simulink model "xactive_rectifier_modified_CSVPWM_22march2025"  (R2024b)
settings: Solver=ode4  StartTime=0.0  StopTime=0.5  FixedStep=1e-6  RelTol=1e-3
values from neighbouring files (symbols this model uses):
  Cdc = 300e-6    (= 0.0003)    [ravi_active_rectifier.m]
  L = 2*Vm/(10000*pi*Ilrms)    (= 0.00173267748608)    [ravi_active_rectifier.m]
  MI = 2*sqrt(2)*Vnphrms/Vdc    [ravi_active_rectifier.m]
  MIL = 2*sqrt(2)*Vm/Vdc    [ravi_active_rectifier.m]
  R = Xl/10    (= 0.0544336686132)    [ravi_active_rectifier.m]
  Vdc = 700    [ravi_active_rectifier.m]
  Vm = 230    [ravi_active_rectifier.m]
libraries: spsIGBTDiodeLib x24, spsThreePhaseVIMeasurementLib x10, spsCurrentMeasurementLib x6, spsVoltageMeasurementLib x6, spsGroundLib x4, spsMeanLib x4, spsPower3phInstantaneousLib x4, simulink x4, spsThreePhaseSeriesRLCBranchLib x3, spsThreePhaseSourceLib x3, spsDCVoltageSourceLib x2, spsSeriesRLCBranchLib x2
settings Model: Creator=Atif iitb  LastModifiedBy=adity
settings DataIOCC: InspectSignalLogs=on  LoggingToFile=on

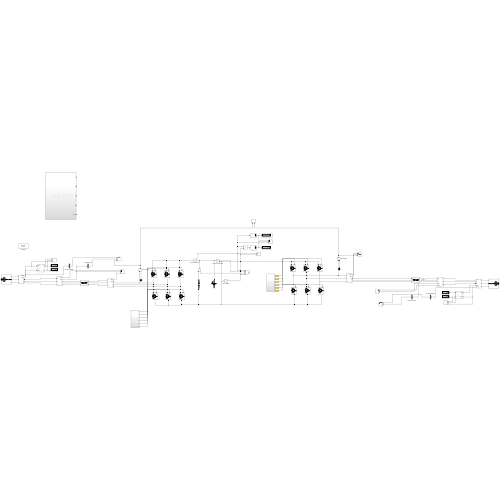
[thumbnail: Simulink's stored preview of the top-level diagram]
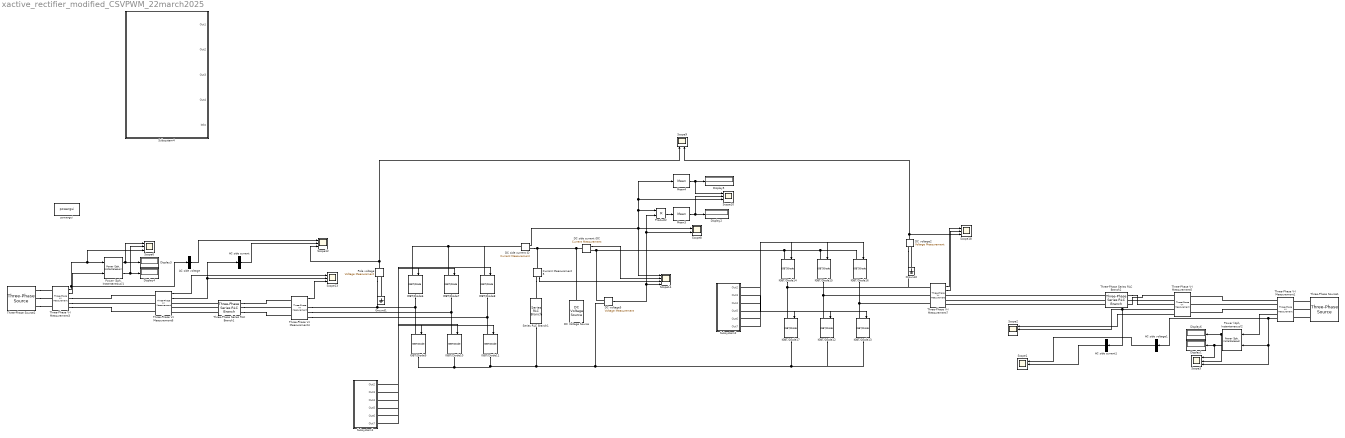
== system xactive_rectifier_modified_CSVPWM_22march2025 ==
  AC side current : Demux  Outputs=3
  AC side current1 : Demux  Outputs=3
  AC side voltage : Demux  Outputs=3
  AC side voltage1 : Demux  Outputs=3
  Current Measurement5 : spsCurrentMeasurementLib/Current Measurement  PhasorSimulation=off  OutputType=Complex  PSBequivalent=0
  DC Voltage Source : spsDCVoltageSourceLib/DC Voltage Source  Amplitude=Vdc  Measurements=None
  DC side current iD : spsCurrentMeasurementLib/Current Measurement  PhasorSimulation=off  OutputType=Complex  PSBequivalent=0
  DC side current iDC : spsCurrentMeasurementLib/Current Measurement  PhasorSimulation=off  OutputType=Complex  PSBequivalent=0
  DC voltage2 : spsVoltageMeasurementLib/Voltage Measurement  PhasorSimulation=off  OutputType=Complex  PSBequivalent=0
  DC voltage5 : spsVoltageMeasurementLib/Voltage Measurement  PhasorSimulation=off  OutputType=Complex  PSBequivalent=0
  Display{1..6} (6 alike) : Display
  Ground1 : spsGroundLib/Ground  LConnTagsString=a
  Ground2 : spsGroundLib/Ground  LConnTagsString=a
  IGBT/Diode{6..17} (12 alike) : spsIGBTDiodeLib/IGBT//Diode  Ron=1e-3  Rs=1e5  Cs=inf  Measurements=off
  Mean3 : spsMeanLib/Mean  Freq=50  Vinit=0  Ts=0
  Mean4 : spsMeanLib/Mean  Freq=50  Vinit=0  Ts=0
  Pole voltage : spsVoltageMeasurementLib/Voltage Measurement  PhasorSimulation=off  OutputType=Complex  PSBequivalent=0
  "Power (3ph, Instantaneous)1" : spsPower3phInstantaneousLib/Power (3ph, Instantaneous)
  "Power (3ph, Instantaneous)2" : spsPower3phInstantaneousLib/Power (3ph, Instantaneous)
  Product2 : Product
  Scope{1..3,6,10,12..13,18} (8 alike) : Scope  NumInputPorts=3
  Scope14 : Scope  NumInputPorts=4
  Scope8 : Scope  NumInputPorts=2
  Scope9 : Scope  NumInputPorts=2
  Series RLC Branch1 : spsSeriesRLCBranchLib/Series RLC Branch  LConnTagsString=__new0  RConnTagsString=__new0  BranchType=C  Resistance=1  Inductance=1e-3  SetiL0=off  InitialCurrent=0  Capacitance=Cdc  Setx0=off  InitialVoltage=0  Measurements=None
  Subsystem1 : Subsystem
  Subsystem2 : Subsystem
  Subsystem4 : Subsystem
  Three-Phase Series RLC Branch1 : spsThreePhaseSeriesRLCBranchLib/Three-Phase Series RLC Branch  LConnTagsString=A|B|C  RConnTagsString=A|B|C  BranchType=RL  Resistance=R  Inductance=L  Capacitance=1e-6  Measurements=None
  Three-Phase Series RLC Branch2 : spsThreePhaseSeriesRLCBranchLib/Three-Phase Series RLC Branch  LConnTagsString=A|B|C  RConnTagsString=A|B|C  BranchType=RL  Resistance=R  Inductance=L  Capacitance=1e-6  Measurements=None
  Three-Phase V-I Measurement1 : spsThreePhaseVIMeasurementLib/Three-Phase V-I Measurement  VoltageMeasurement=phase-to-ground  SetLabelV=off  LabelV=Vabc  Vpu=off  VpuLL=off  CurrentMeasurement=yes  SetLabelI=off  LabelI=Iabc  Ipu=off  Pbase=100e6  Vbase=500e3  OutputType=Complex  PhasorSimulation=off  PSBequivalent=0
  Three-Phase V-I Measurement3 : spsThreePhaseVIMeasurementLib/Three-Phase V-I Measurement  VoltageMeasurement=phase-to-ground  SetLabelV=off  LabelV=Vabc  Vpu=off  VpuLL=off  CurrentMeasurement=yes  SetLabelI=off  LabelI=Iabc  Ipu=off  Pbase=100e6  Vbase=500e3  OutputType=Complex  PhasorSimulation=off  PSBequivalent=0
  Three-Phase V-I Measurement4 : spsThreePhaseVIMeasurementLib/Three-Phase V-I Measurement  VoltageMeasurement=phase-to-phase  SetLabelV=off  LabelV=Vabc  Vpu=off  VpuLL=off  CurrentMeasurement=yes  SetLabelI=off  LabelI=Iabc  Ipu=off  Pbase=100e6  Vbase=500e3  OutputType=Complex  PhasorSimulation=off  PSBequivalent=0
  Three-Phase V-I Measurement5 : spsThreePhaseVIMeasurementLib/Three-Phase V-I Measurement  VoltageMeasurement=phase-to-phase  SetLabelV=off  LabelV=Vabc  Vpu=off  VpuLL=off  CurrentMeasurement=yes  SetLabelI=off  LabelI=Iabc  Ipu=off  Pbase=100e6  Vbase=500e3  OutputType=Complex  PhasorSimulation=off  PSBequivalent=0
  Three-Phase V-I Measurement6 : spsThreePhaseVIMeasurementLib/Three-Phase V-I Measurement  VoltageMeasurement=phase-to-phase  SetLabelV=off  LabelV=Vabc  Vpu=off  VpuLL=off  CurrentMeasurement=yes  SetLabelI=off  LabelI=Iabc  Ipu=off  Pbase=100e6  Vbase=500e3  OutputType=Complex  PhasorSimulation=off  PSBequivalent=0
  Three-Phase V-I Measurement7 : spsThreePhaseVIMeasurementLib/Three-Phase V-I Measurement  VoltageMeasurement=phase-to-ground  SetLabelV=off  LabelV=Vabc  Vpu=off  VpuLL=off  CurrentMeasurement=yes  SetLabelI=off  LabelI=Iabc  Ipu=off  Pbase=100e6  Vbase=500e3  OutputType=Complex  PhasorSimulation=off  PSBequivalent=0
  Three-Phase Source1 : spsThreePhaseSourceLib/Three-Phase Source  InternalConnection=Yg  VoltagePhases=off  Voltage=2.335782132615092e+02*sqrt(3)  PhaseAngle=0.890192885516744  Voltage_phases=[25e3 25e3 25e3]/sqrt(3)  PhaseAngles_phases=[0 -120 +120]  Frequency=50  NonIdealSource=off  SpecifyImpedance=off  Resistance=0.8929  Inductance=16.58e-3  ShortCircuitLevel=100e6  BaseVoltage=25e3  XRratio=7  BusType=swing  Pref=10e3  Qref=0  Prefabc=[10e3, 10e3, 10e3]  Qrefabc=[0, 0, 0]  Qmin=-inf  Qmax=inf
  Three-Phase Source2 : spsThreePhaseSourceLib/Three-Phase Source  InternalConnection=Yg  VoltagePhases=off  Voltage=Vm*sqrt(3)  PhaseAngle=Delta  Voltage_phases=[25e3 25e3 25e3]/sqrt(3)  PhaseAngles_phases=[0 -120 +120]  Frequency=50  NonIdealSource=off  SpecifyImpedance=off  Resistance=0.8929  Inductance=16.58e-3  ShortCircuitLevel=100e6  BaseVoltage=25e3  XRratio=7  BusType=swing  Pref=10e3  Qref=0  Prefabc=[10e3, 10e3, 10e3]  Qrefabc=[0, 0, 0]  Qmin=-inf  Qmax=inf
  powergui : sps_lib/powergui  Priority=1  SimulationMode=Discrete  SampleTime=1e-6  frequency=60  Iterations=50  frequencyindice=0  Pbase=100e6  ErrMax=1e-4  UnitsV=kV  UnitsW=MW  buscounter=0  FunctionMessages=off  echomessages=off  EnableUseOfTLC=off  CurrentSourceSwitches=off  DisableSnubberDevices=off  DisableRonSwitches=off  DisableVfSwitches=off  DisplayEquations=off  AutomaticDiscreteSolvers=off  SolverType=Tustin/Backward Euler (TBE)  Interpol=off  ExternalGateDelay=off  methode=off  Ts=100  x0status=blocks  SPID=on  SwTol=0  HookPort=off  NonlinearTolerance=1e-4  nMaxIteration=100  ContinueOnMaxIteration=off  RestoreLinks=warning  ResistiveCurrentMeasurement=off  Frange=[0:2:500]  Ylog=off  Xlog=on  ShowGrid=off  save=off  variable=ZData  structure=0  ZoomFFT=off  StartTime=0.0  cycles=1  DisplayStyle=1  fundamental=60  FreqAxis=off  MaxFrequency=1000  frequencyindicesteady=1  RmsSteady=1  display=off
  wires:
  Subsystem1/2(Out3) -> IGBT/Diode9/1
  Subsystem1/6(Out7) -> IGBT/Diode11/1
  Mean4/1 -> Scope10/1, Display5/1
  Subsystem1/3(Out4) -> IGBT/Diode7/1
  DC side current iD/1 -> Scope14/1, Mean4/1, Scope10/3, Product2/1, Scope8/1
  Subsystem1/5(Out6) -> IGBT/Diode8/1
  AC side current/2 -> Scope12/2
  Mean3/1 -> Scope10/2, Display2/1
  Three-Phase V-I Measurement6/2 -> Scope13/2, AC side current/1
  Product2/1 -> Mean3/1
  Three-Phase V-I Measurement4/1 -> Scope13/3
  Subsystem1/1(Out2) -> IGBT/Diode6/1
  Pole voltage/1 -> Scope12/3, Scope9/1
  Three-Phase V-I Measurement6/1 -> Scope13/1
  Subsystem1/4(Out5) -> IGBT/Diode10/1
  Three-Phase V-I Measurement3/1 -> AC side voltage/1, Scope6/3, "Power (3ph, Instantaneous)1"/1
  Three-Phase V-I Measurement3/2 -> "Power (3ph, Instantaneous)1"/2
  "Power (3ph, Instantaneous)1"/1 -> Scope6/1, Display3/1
  "Power (3ph, Instantaneous)1"/2 -> Scope6/2, Display4/1
  AC side voltage/2 -> Scope12/1
  DC voltage5/1 -> Scope8/2, Product2/2, Scope14/4
  Current Measurement5/1 -> Scope14/3
  DC side current iDC/1 -> Scope14/2
  Subsystem2/1(Out2) -> IGBT/Diode14/1
  Subsystem2/2(Out3) -> IGBT/Diode17/1
  Subsystem2/3(Out4) -> IGBT/Diode15/1
  Subsystem2/4(Out5) -> IGBT/Diode12/1
  Subsystem2/5(Out6) -> IGBT/Diode16/1
  Subsystem2/6(Out7) -> IGBT/Diode13/1
  Three-Phase V-I Measurement7/2 -> Scope18/2
  Three-Phase V-I Measurement7/1 -> Scope18/1
  DC voltage2/1 -> Scope18/3, Scope9/2
  AC side voltage1/2 -> Scope1/1
  Three-Phase V-I Measurement1/1 -> Scope3/3, "Power (3ph, Instantaneous)2"/1, AC side voltage1/1
  "Power (3ph, Instantaneous)2"/2 -> Scope3/2, Display6/1
  Three-Phase V-I Measurement1/2 -> "Power (3ph, Instantaneous)2"/2
  AC side current1/2 -> Scope1/2
  Three-Phase V-I Measurement5/1 -> Scope2/1
  Three-Phase V-I Measurement5/2 -> Scope2/2, AC side current1/1
  "Power (3ph, Instantaneous)2"/1 -> Scope3/1, Display1/1
  connections:
  Pole voltage/LConn1 -- Three-Phase V-I Measurement4/RConn1 -- IGBT/Diode6/RConn1 -- IGBT/Diode9/LConn1
  IGBT/Diode6/LConn1 -- IGBT/Diode7/LConn1 -- IGBT/Diode8/LConn1 -- DC side current iD/LConn1
  Three-Phase V-I Measurement4/RConn2 -- IGBT/Diode7/RConn1 -- IGBT/Diode10/LConn1
  Three-Phase V-I Measurement4/RConn3 -- IGBT/Diode8/RConn1 -- IGBT/Diode11/LConn1
  Three-Phase Series RLC Branch1/RConn1 -- Three-Phase V-I Measurement4/LConn1
  Three-Phase Series RLC Branch1/LConn1 -- Three-Phase V-I Measurement6/RConn1
  Three-Phase Series RLC Branch1/RConn2 -- Three-Phase V-I Measurement4/LConn2
  Three-Phase Series RLC Branch1/RConn3 -- Three-Phase V-I Measurement4/LConn3
  Three-Phase Series RLC Branch1/LConn2 -- Three-Phase V-I Measurement6/RConn2
  Three-Phase Series RLC Branch1/LConn3 -- Three-Phase V-I Measurement6/RConn3
  Three-Phase Source2/RConn1 -- Three-Phase V-I Measurement3/LConn1
  Three-Phase Source2/RConn2 -- Three-Phase V-I Measurement3/LConn2
  Three-Phase Source2/RConn3 -- Three-Phase V-I Measurement3/LConn3
  Three-Phase V-I Measurement3/RConn1 -- Three-Phase V-I Measurement6/LConn1
  Three-Phase V-I Measurement3/RConn2 -- Three-Phase V-I Measurement6/LConn2
  Three-Phase V-I Measurement3/RConn3 -- Three-Phase V-I Measurement6/LConn3
  Current Measurement5/RConn1 -- Series RLC Branch1/LConn1
  DC side current iD/RConn1 -- Current Measurement5/LConn1 -- DC Voltage Source/RConn1 -- DC side current iDC/LConn1
  IGBT/Diode15/RConn1 -- Three-Phase V-I Measurement7/LConn2 -- IGBT/Diode12/LConn1
  IGBT/Diode14/RConn1 -- DC voltage2/LConn1 -- Three-Phase V-I Measurement7/LConn1 -- IGBT/Diode17/LConn1
  IGBT/Diode16/RConn1 -- Three-Phase V-I Measurement7/LConn3 -- IGBT/Diode13/LConn1
  DC side current iDC/RConn1 -- IGBT/Diode14/LConn1 -- IGBT/Diode15/LConn1 -- IGBT/Diode16/LConn1 -- DC voltage5/LConn1
  Ground1/LConn1 -- Pole voltage/LConn2
  Ground2/LConn1 -- DC voltage2/LConn2
  IGBT/Diode9/RConn1 -- Series RLC Branch1/RConn1 -- IGBT/Diode12/RConn1 -- IGBT/Diode13/RConn1 -- IGBT/Diode17/RConn1 -- DC voltage5/LConn2 -- IGBT/Diode11/RConn1 -- IGBT/Diode10/RConn1
  Three-Phase Series RLC Branch2/LConn2 -- Three-Phase V-I Measurement5/RConn2
  Three-Phase Source1/RConn3 -- Three-Phase V-I Measurement1/LConn3
  Three-Phase Source1/RConn1 -- Three-Phase V-I Measurement1/LConn1
  Three-Phase Source1/RConn2 -- Three-Phase V-I Measurement1/LConn2
  Three-Phase Series RLC Branch2/LConn1 -- Three-Phase V-I Measurement5/RConn1
  Three-Phase V-I Measurement1/RConn3 -- Three-Phase V-I Measurement5/LConn3
  Three-Phase V-I Measurement1/RConn1 -- Three-Phase V-I Measurement5/LConn1
  Three-Phase Series RLC Branch2/LConn3 -- Three-Phase V-I Measurement5/RConn3
  Three-Phase V-I Measurement1/RConn2 -- Three-Phase V-I Measurement5/LConn2
  Three-Phase Series RLC Branch2/RConn1 -- Three-Phase V-I Measurement7/RConn1
  Three-Phase Series RLC Branch2/RConn2 -- Three-Phase V-I Measurement7/RConn2
  Three-Phase Series RLC Branch2/RConn3 -- Three-Phase V-I Measurement7/RConn3

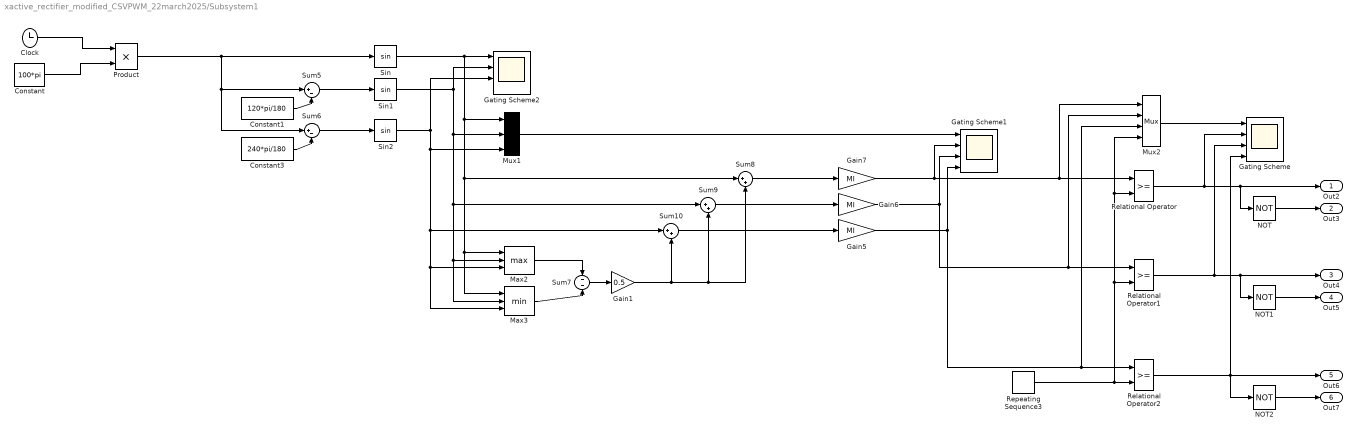
== system xactive_rectifier_modified_CSVPWM_22march2025/Subsystem1 ==
  Clock : Clock
  Constant : Constant  Value=100*pi
  Constant1 : Constant  Value=120*pi/180
  Constant3 : Constant  Value=240*pi/180
  Gain1 : Gain  Gain=0.5
  Gain5 : Gain  Gain=MI
  Gain6 : Gain  Gain=MI
  Gain7 : Gain  Gain=MI
  Gating Scheme : Scope  NumInputPorts=4
  Gating Scheme1 : Scope  NumInputPorts=4
  Gating Scheme2 : Scope  NumInputPorts=4
  Max2 : MinMax  Function=max  Inputs=3
  Max3 : MinMax  Inputs=3
  Mux1 : Mux  Inputs=3.
  Mux2 : Mux
  NOT : Logic  Operator=NOT  IconShape=distinctive  AllPortsSameDT=off  OutDataTypeStr=boolean
  NOT1 : Logic  Operator=NOT  IconShape=distinctive  AllPortsSameDT=off  OutDataTypeStr=boolean
  NOT2 : Logic  Operator=NOT  IconShape=distinctive  AllPortsSameDT=off  OutDataTypeStr=boolean
  Product : Product
  Relational Operator : RelationalOperator  OutDataTypeStr=boolean  RndMeth=Simplest  InputSameDT=off
  Relational Operator1 : RelationalOperator  OutDataTypeStr=boolean  RndMeth=Simplest  InputSameDT=off
  Relational Operator2 : RelationalOperator  OutDataTypeStr=boolean  RndMeth=Simplest  InputSameDT=off
  Repeating Sequence3 : simulink/Sources/Repeating Sequence  rep_seq_t=[0 1 2]*[1/40000]  rep_seq_y=[-1 1 -1]
  Sin : Trigonometry
  Sin1 : Trigonometry
  Sin2 : Trigonometry
  Sum10 : Sum  Inputs=|++
  Sum5 : Sum  Inputs=|+-
  Sum6 : Sum  Inputs=|+-
  Sum7 : Sum  Inputs=--
  Sum8 : Sum  Inputs=|++
  Sum9 : Sum  Inputs=|++
  Out2 : Outport
  Out3 : Outport  Port=2
  Out4 : Outport  Port=3
  Out5 : Outport  Port=4
  Out6 : Outport  Port=5
  Out7 : Outport  Port=6
  wires:
  NOT2/1 -> Out7/1
  Constant/1 -> Product/2
  Constant1/1 -> Sum5/2
  Sin/1 -> Gating Scheme2/1, Sum8/1, Max2/1, Max3/1, Mux1/1
  Relational Operator2/1 -> Out6/1, Gating Scheme/4, NOT2/1
  Sum10/1 -> Gain5/1
  NOT/1 -> Out3/1
  Relational Operator/1 -> Out2/1, NOT/1, Gating Scheme/2
  Sum9/1 -> Gain6/1
  Sum5/1 -> Sin1/1
  Product/1 -> Sin/1, Sum6/1, Sum5/1
  Mux2/1 -> Gating Scheme/1
  Sin2/1 -> Sum10/1, Max3/3, Max2/3, Mux1/3, Gating Scheme2/3
  Sin1/1 -> Max3/2, Max2/2, Sum9/1, Mux1/2, Gating Scheme2/2
  Clock/1 -> Product/1
  Repeating Sequence3/1 -> Relational Operator1/2, Mux2/4, Relational Operator/2, Relational Operator2/2
  Relational Operator1/1 -> Out4/1, NOT1/1, Gating Scheme/3
  Max2/1 -> Sum7/1
  Sum7/1 -> Gain1/1
  Max3/1 -> Sum7/2
  Constant3/1 -> Sum6/2
  Sum6/1 -> Sin2/1
  NOT1/1 -> Out5/1
  Mux1/1 -> Gating Scheme1/1
  Gain1/1 -> Sum10/2, Sum9/2, Sum8/2
  Sum8/1 -> Gain7/1
  Gain7/1 -> Gating Scheme1/2, Mux2/1, Relational Operator/1
  Gain6/1 -> Mux2/2, Relational Operator1/1, Gating Scheme1/3
  Gain5/1 -> Mux2/3, Relational Operator2/1, Gating Scheme1/4

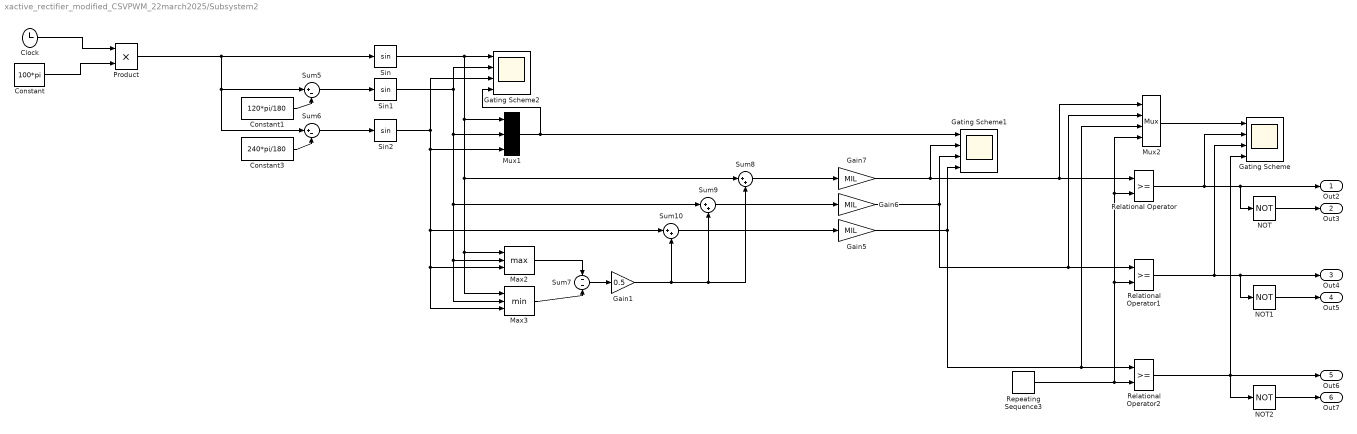
== system xactive_rectifier_modified_CSVPWM_22march2025/Subsystem2 ==
  Clock : Clock
  Constant : Constant  Value=100*pi
  Constant1 : Constant  Value=120*pi/180
  Constant3 : Constant  Value=240*pi/180
  Gain1 : Gain  Gain=0.5
  Gain5 : Gain  Gain=MIL
  Gain6 : Gain  Gain=MIL
  Gain7 : Gain  Gain=MIL
  Gating Scheme : Scope  NumInputPorts=4
  Gating Scheme1 : Scope  NumInputPorts=4
  Gating Scheme2 : Scope  NumInputPorts=4
  Max2 : MinMax  Function=max  Inputs=3
  Max3 : MinMax  Inputs=3
  Mux1 : Mux  Inputs=3.
  Mux2 : Mux
  NOT : Logic  Operator=NOT  IconShape=distinctive  AllPortsSameDT=off  OutDataTypeStr=boolean
  NOT1 : Logic  Operator=NOT  IconShape=distinctive  AllPortsSameDT=off  OutDataTypeStr=boolean
  NOT2 : Logic  Operator=NOT  IconShape=distinctive  AllPortsSameDT=off  OutDataTypeStr=boolean
  Product : Product
  Relational Operator : RelationalOperator  OutDataTypeStr=boolean  RndMeth=Simplest  InputSameDT=off
  Relational Operator1 : RelationalOperator  OutDataTypeStr=boolean  RndMeth=Simplest  InputSameDT=off
  Relational Operator2 : RelationalOperator  OutDataTypeStr=boolean  RndMeth=Simplest  InputSameDT=off
  Repeating Sequence3 : simulink/Sources/Repeating Sequence  rep_seq_t=[0 1 2]*[1/40000]  rep_seq_y=[-1 1 -1]
  Sin : Trigonometry
  Sin1 : Trigonometry
  Sin2 : Trigonometry
  Sum10 : Sum  Inputs=|++
  Sum5 : Sum  Inputs=|+-
  Sum6 : Sum  Inputs=|+-
  Sum7 : Sum  Inputs=--
  Sum8 : Sum  Inputs=|++
  Sum9 : Sum  Inputs=|++
  Out2 : Outport
  Out3 : Outport  Port=2
  Out4 : Outport  Port=3
  Out5 : Outport  Port=4
  Out6 : Outport  Port=5
  Out7 : Outport  Port=6
  wires:
  Gain5/1 -> Gating Scheme1/4, Relational Operator2/1, Mux2/3
  Gain6/1 -> Gating Scheme1/3, Relational Operator1/1, Mux2/2
  Gain7/1 -> Relational Operator/1, Mux2/1, Gating Scheme1/2
  Sum8/1 -> Gain7/1
  Gain1/1 -> Sum8/2, Sum9/2, Sum10/2
  Mux1/1 -> Gating Scheme2/4, Gating Scheme1/1
  NOT1/1 -> Out5/1
  Sum6/1 -> Sin2/1
  Constant3/1 -> Sum6/2
  Max3/1 -> Sum7/2
  Sum7/1 -> Gain1/1
  Max2/1 -> Sum7/1
  Relational Operator1/1 -> Gating Scheme/3, NOT1/1, Out4/1
  Repeating Sequence3/1 -> Relational Operator2/2, Relational Operator/2, Mux2/4, Relational Operator1/2
  Clock/1 -> Product/1
  Sin1/1 -> Gating Scheme2/2, Mux1/2, Sum9/1, Max2/2, Max3/2
  Sin2/1 -> Gating Scheme2/3, Mux1/3, Max2/3, Max3/3, Sum10/1
  Mux2/1 -> Gating Scheme/1
  Product/1 -> Sum5/1, Sum6/1, Sin/1
  Sum5/1 -> Sin1/1
  Sum9/1 -> Gain6/1
  Relational Operator/1 -> Gating Scheme/2, NOT/1, Out2/1
  NOT/1 -> Out3/1
  Sum10/1 -> Gain5/1
  Relational Operator2/1 -> NOT2/1, Gating Scheme/4, Out6/1
  Sin/1 -> Mux1/1, Max3/1, Max2/1, Sum8/1, Gating Scheme2/1
  Constant1/1 -> Sum5/2
  Constant/1 -> Product/2
  NOT2/1 -> Out7/1

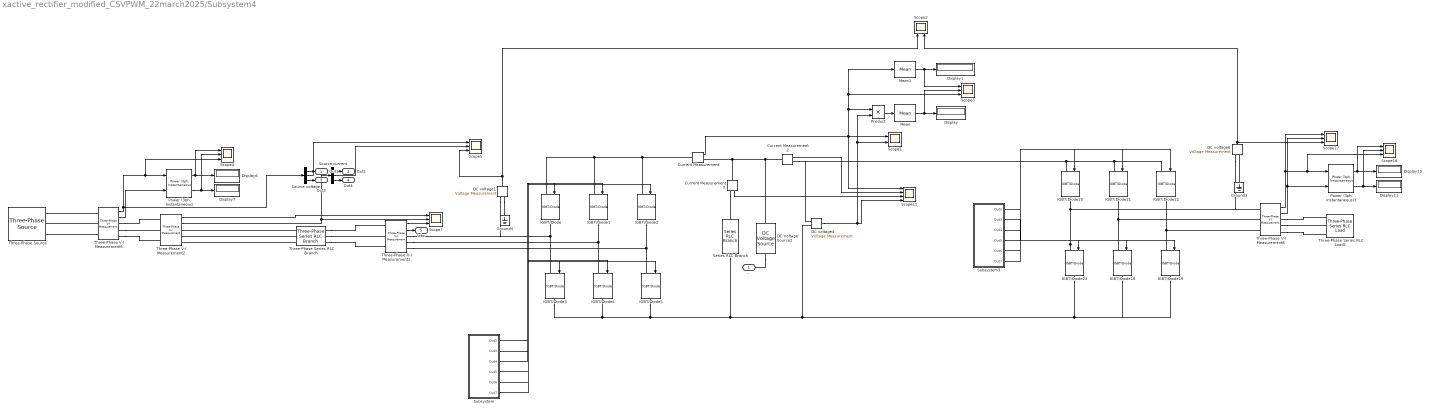
== system xactive_rectifier_modified_CSVPWM_22march2025/Subsystem4 ==
  Current Measurement : spsCurrentMeasurementLib/Current Measurement  PhasorSimulation=off  OutputType=Complex  PSBequivalent=0
  Current Measurement2 : spsCurrentMeasurementLib/Current Measurement  PhasorSimulation=off  OutputType=Complex  PSBequivalent=0
  Current Measurement3 : spsCurrentMeasurementLib/Current Measurement  PhasorSimulation=off  OutputType=Complex  PSBequivalent=0
  DC Voltage Source2 : spsDCVoltageSourceLib/DC Voltage Source  Amplitude=Vdc  Measurements=None
  DC voltage1 : spsVoltageMeasurementLib/Voltage Measurement  PhasorSimulation=off  OutputType=Complex  PSBequivalent=0
  DC voltage4 : spsVoltageMeasurementLib/Voltage Measurement  PhasorSimulation=off  OutputType=Complex  PSBequivalent=0
  DC voltage6 : spsVoltageMeasurementLib/Voltage Measurement  PhasorSimulation=off  OutputType=Complex  PSBequivalent=0
  Display{,1,6..7,10..11} (6 alike) : Display
  Ground3 : spsGroundLib/Ground  LConnTagsString=a
  Ground4 : spsGroundLib/Ground  LConnTagsString=a
  IGBT/Diode{,1..5,18..23} (12 alike) : spsIGBTDiodeLib/IGBT//Diode  Ron=1e-3  Rs=1e5  Cs=inf  Measurements=off
  Mean : spsMeanLib/Mean  Freq=50  Vinit=0  Ts=0
  Mean1 : spsMeanLib/Mean  Freq=50  Vinit=0  Ts=0
  "Power (3ph, Instantaneous)" : spsPower3phInstantaneousLib/Power (3ph, Instantaneous)
  "Power (3ph, Instantaneous)3" : spsPower3phInstantaneousLib/Power (3ph, Instantaneous)
  Product : Product
  Scope1 : Scope  NumInputPorts=2
  Scope11 : Scope  NumInputPorts=4
  Scope{3..5,7,16..17} (6 alike) : Scope  NumInputPorts=3
  Scope2 : Scope  NumInputPorts=2
  Series RLC Branch : spsSeriesRLCBranchLib/Series RLC Branch  LConnTagsString=__new0  RConnTagsString=__new0  BranchType=C  Resistance=1  Inductance=1e-3  SetiL0=off  InitialCurrent=0  Capacitance=Cdc  Setx0=off  InitialVoltage=0  Measurements=None
  Source current : Demux  Outputs=3
  Source voltage : Demux  Outputs=3
  Subsystem : Subsystem
  Subsystem3 : Subsystem
  Three-Phase Series RLC Branch : spsThreePhaseSeriesRLCBranchLib/Three-Phase Series RLC Branch  LConnTagsString=A|B|C  RConnTagsString=A|B|C  BranchType=RL  Resistance=R  Inductance=L  Capacitance=1e-6  Measurements=None
  Three-Phase Series RLC Load1 : spsThreePhaseSeriesRLCLoadLib/Three-Phase Series RLC Load  LConnTagsString=A|B|C  Configuration=Y (grounded)  NominalVoltage=230*sqrt(3)  Vabc=[1e3 1e3 1e3]  Vabcp=[1e3 1e3 1e3]  NominalFrequency=50  UnbalancedPower=off  ActivePower=0  InductivePower=QL  CapacitivePower=0  Pabc=[10e3 9e3 11e3]  QLabc=[100 90 110]  QCabc=[100 90 110]  Pabcp=[10e3 9e3 11e3]  QLabcp=[100 90 110]  QCabcp=[100 90 110]  Measurements=None  LoadType=constant Z
  Three-Phase V-I Measurement{1..2,5,8} (4 alike) : spsThreePhaseVIMeasurementLib/Three-Phase V-I Measurement  VoltageMeasurement=phase-to-ground  SetLabelV=off  LabelV=Vabc  Vpu=off  VpuLL=off  CurrentMeasurement=yes  SetLabelI=off  LabelI=Iabc  Ipu=off  Pbase=100e6  Vbase=500e3  OutputType=Complex  PhasorSimulation=off  PSBequivalent=0
  Three-Phase Source : spsThreePhaseSourceLib/Three-Phase Source  InternalConnection=Yg  VoltagePhases=off  Voltage=Vm*sqrt(3)  PhaseAngle=Delta  Voltage_phases=[25e3 25e3 25e3]/sqrt(3)  PhaseAngles_phases=[0 -120 +120]  Frequency=50  NonIdealSource=off  SpecifyImpedance=off  Resistance=0.8929  Inductance=16.58e-3  ShortCircuitLevel=100e6  BaseVoltage=25e3  XRratio=7  BusType=swing  Pref=10e3  Qref=0  Prefabc=[10e3, 10e3, 10e3]  Qrefabc=[0, 0, 0]  Qmin=-inf  Qmax=inf
  - : PMIOPort  Side=Left
  Out1 : Outport
  Out2 : Outport  Port=2
  Out3 : Outport  Port=3
  Out4 : Outport  Port=4
  Iabc : Outport  Port=5
  wires:
  Subsystem/4(Out5) -> IGBT/Diode4/1
  Subsystem/5(Out6) -> IGBT/Diode2/1
  Current Measurement/1 -> Scope11/1, Mean1/1, Scope3/3, Product/1, Scope1/1
  "Power (3ph, Instantaneous)3"/1 -> Display10/1, Scope16/1
  DC voltage6/1 -> Scope2/2, Scope17/3
  Three-Phase V-I Measurement2/1 -> Scope7/1
  Subsystem3/2(Out3) -> IGBT/Diode23/1
  Source voltage/2 -> Scope5/1
  Current Measurement2/1 -> Scope11/2
  Subsystem3/6(Out7) -> IGBT/Diode19/1
  Subsystem/3(Out4) -> IGBT/Diode1/1
  Three-Phase V-I Measurement5/1 -> Source voltage/1, Scope4/3, "Power (3ph, Instantaneous)"/1
  Subsystem/1(Out2) -> IGBT/Diode/1
  Three-Phase V-I Measurement8/1 -> Scope17/1, "Power (3ph, Instantaneous)3"/1, Scope16/3
  Three-Phase V-I Measurement2/2 -> Source current/1, Scope7/2
  Three-Phase V-I Measurement8/2 -> Scope17/2, "Power (3ph, Instantaneous)3"/2
  Subsystem3/4(Out5) -> IGBT/Diode18/1
  Mean1/1 -> Scope3/1, Display1/1
  Product/1 -> Mean/1
  "Power (3ph, Instantaneous)3"/2 -> Display11/1, Scope16/2
  Three-Phase V-I Measurement5/2 -> "Power (3ph, Instantaneous)"/2
  Three-Phase V-I Measurement1/2 -> Iabc/1
  Source current/2 -> Scope5/2
  Subsystem/6(Out7) -> IGBT/Diode5/1
  Subsystem3/5(Out6) -> IGBT/Diode22/1
  Source voltage/1 -> Out1/1
  DC voltage1/1 -> Scope5/3, Scope2/1
  Subsystem3/3(Out4) -> IGBT/Diode21/1
  "Power (3ph, Instantaneous)"/1 -> Scope4/1, Display6/1
  Subsystem/2(Out3) -> IGBT/Diode3/1
  Subsystem3/1(Out2) -> IGBT/Diode20/1
  Three-Phase V-I Measurement1/1 -> Scope7/3
  Current Measurement3/1 -> Scope11/3
  "Power (3ph, Instantaneous)"/2 -> Scope4/2, Display7/1
  DC voltage4/1 -> Product/2, Scope1/2, Scope11/4
  Mean/1 -> Scope3/2, Display/1
  Source current/1 -> Out2/1
  Source voltage/3 -> Out3/1
  Source current/3 -> Out4/1
  connections:
  Current Measurement3/LConn1 -- Current Measurement2/LConn1 -- DC Voltage Source2/RConn1 -- Current Measurement/RConn1
  IGBT/Diode22/RConn1 -- Three-Phase V-I Measurement8/LConn3 -- IGBT/Diode19/LConn1
  Three-Phase V-I Measurement5/RConn2 -- Three-Phase V-I Measurement2/LConn2
  Three-Phase V-I Measurement8/RConn2 -- Three-Phase Series RLC Load1/LConn2
  IGBT/Diode5/RConn1 -- Series RLC Branch/RConn1 -- IGBT/Diode23/RConn1 -- IGBT/Diode18/RConn1 -- IGBT/Diode19/RConn1 -- DC voltage4/LConn2 -- IGBT/Diode4/RConn1 -- IGBT/Diode3/RConn1
  Three-Phase V-I Measurement5/RConn3 -- Three-Phase V-I Measurement2/LConn3
  Three-Phase V-I Measurement5/LConn3 -- Three-Phase Source/RConn3
  Three-Phase Series RLC Branch/RConn2 -- Three-Phase V-I Measurement1/LConn2
  IGBT/Diode2/LConn1 -- IGBT/Diode/LConn1 -- IGBT/Diode1/LConn1 -- Current Measurement/LConn1
  IGBT/Diode20/LConn1 -- DC voltage4/LConn1 -- Current Measurement2/RConn1 -- IGBT/Diode21/LConn1 -- IGBT/Diode22/LConn1
  DC voltage1/LConn2 -- Ground4/LConn1
  DC Voltage Source2/LConn1 -- -/RConn1
  IGBT/Diode/RConn1 -- Three-Phase V-I Measurement1/RConn1 -- DC voltage1/LConn1 -- IGBT/Diode3/LConn1
  Three-Phase V-I Measurement8/RConn3 -- Three-Phase Series RLC Load1/LConn3
  Three-Phase V-I Measurement5/LConn2 -- Three-Phase Source/RConn2
  IGBT/Diode1/RConn1 -- Three-Phase V-I Measurement1/RConn2 -- IGBT/Diode4/LConn1
  Three-Phase Series RLC Branch/LConn3 -- Three-Phase V-I Measurement2/RConn3
  IGBT/Diode23/LConn1 -- DC voltage6/LConn1 -- Three-Phase V-I Measurement8/LConn1 -- IGBT/Diode20/RConn1
  Three-Phase V-I Measurement8/RConn1 -- Three-Phase Series RLC Load1/LConn1
  Three-Phase V-I Measurement5/LConn1 -- Three-Phase Source/RConn1
  Three-Phase Series RLC Branch/LConn2 -- Three-Phase V-I Measurement2/RConn2
  Three-Phase V-I Measurement5/RConn1 -- Three-Phase V-I Measurement2/LConn1
  Three-Phase Series RLC Branch/RConn1 -- Three-Phase V-I Measurement1/LConn1
  Current Measurement3/RConn1 -- Series RLC Branch/LConn1
  Three-Phase Series RLC Branch/RConn3 -- Three-Phase V-I Measurement1/LConn3
  IGBT/Diode21/RConn1 -- Three-Phase V-I Measurement8/LConn2 -- IGBT/Diode18/LConn1
  Ground3/LConn1 -- DC voltage6/LConn2
  IGBT/Diode2/RConn1 -- Three-Phase V-I Measurement1/RConn3 -- IGBT/Diode5/LConn1
  Three-Phase Series RLC Branch/LConn1 -- Three-Phase V-I Measurement2/RConn1

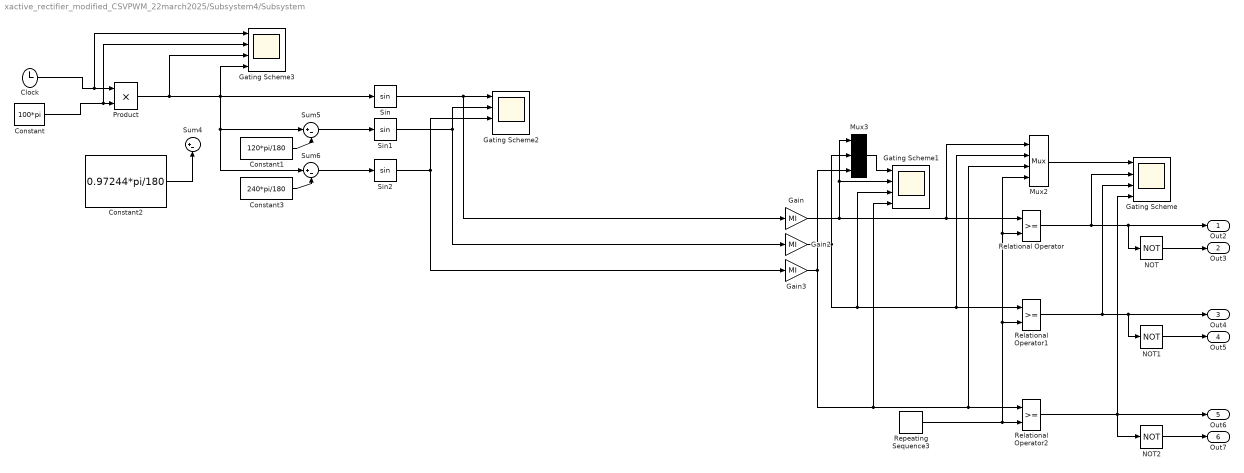
== system xactive_rectifier_modified_CSVPWM_22march2025/Subsystem4/Subsystem ==
  Clock : Clock
  Constant : Constant  Value=100*pi
  Constant1 : Constant  Value=120*pi/180
  Constant2 : Constant  Value=0.97244*pi/180
  Constant3 : Constant  Value=240*pi/180
  Gain : Gain  Gain=MI
  Gain2 : Gain  Gain=MI
  Gain3 : Gain  Gain=MI
  Gating Scheme{,1..3} (4 alike) : Scope  NumInputPorts=4
  Mux2 : Mux
  Mux3 : Mux  Inputs=3.
  NOT : Logic  Operator=NOT  IconShape=distinctive  AllPortsSameDT=off  OutDataTypeStr=boolean
  NOT1 : Logic  Operator=NOT  IconShape=distinctive  AllPortsSameDT=off  OutDataTypeStr=boolean
  NOT2 : Logic  Operator=NOT  IconShape=distinctive  AllPortsSameDT=off  OutDataTypeStr=boolean
  Product : Product
  Relational Operator : RelationalOperator  OutDataTypeStr=boolean  RndMeth=Simplest  InputSameDT=off
  Relational Operator1 : RelationalOperator  OutDataTypeStr=boolean  RndMeth=Simplest  InputSameDT=off
  Relational Operator2 : RelationalOperator  OutDataTypeStr=boolean  RndMeth=Simplest  InputSameDT=off
  Repeating Sequence3 : simulink/Sources/Repeating Sequence  rep_seq_t=[0 1 2]*[1/10000]  rep_seq_y=[-1 1 -1]
  Sin : Trigonometry
  Sin1 : Trigonometry
  Sin2 : Trigonometry
  Sum4 : Sum  Inputs=|+-
  Sum5 : Sum  Inputs=|+-
  Sum6 : Sum  Inputs=|+-
  Out2 : Outport
  Out3 : Outport  Port=2
  Out4 : Outport  Port=3
  Out5 : Outport  Port=4
  Out6 : Outport  Port=5
  Out7 : Outport  Port=6
  wires:
  NOT2/1 -> Out7/1
  Constant/1 -> Gating Scheme3/2, Product/2
  Constant1/1 -> Sum5/2
  Relational Operator2/1 -> Out6/1, Gating Scheme/4, NOT2/1
  Sin2/1 -> Gating Scheme2/3, Gain3/1
  NOT/1 -> Out3/1
  Relational Operator/1 -> Out2/1, NOT/1, Gating Scheme/2
  Sin1/1 -> Gain2/1, Gating Scheme2/2
  Sum5/1 -> Sin1/1
  Product/1 -> Gating Scheme3/4, Sin/1, Sum6/1, Sum5/1, Gating Scheme3/3
  Mux2/1 -> Gating Scheme/1
  Clock/1 -> Gating Scheme3/1, Product/1
  Repeating Sequence3/1 -> Relational Operator1/2, Relational Operator/2, Mux2/4, Relational Operator2/2
  Relational Operator1/1 -> Out4/1, NOT1/1, Gating Scheme/3
  Sin/1 -> Gain/1, Gating Scheme2/1
  Constant3/1 -> Sum6/2
  Sum6/1 -> Sin2/1
  NOT1/1 -> Out5/1
  Gain/1 -> Mux3/1, Gating Scheme1/2, Mux2/1, Relational Operator/1
  Gain2/1 -> Gating Scheme1/3, Mux2/2, Relational Operator1/1, Mux3/2
  Gain3/1 -> Gating Scheme1/4, Mux2/3, Relational Operator2/1, Mux3/3
  Mux3/1 -> Gating Scheme1/1
  Constant2/1 -> Sum4/2

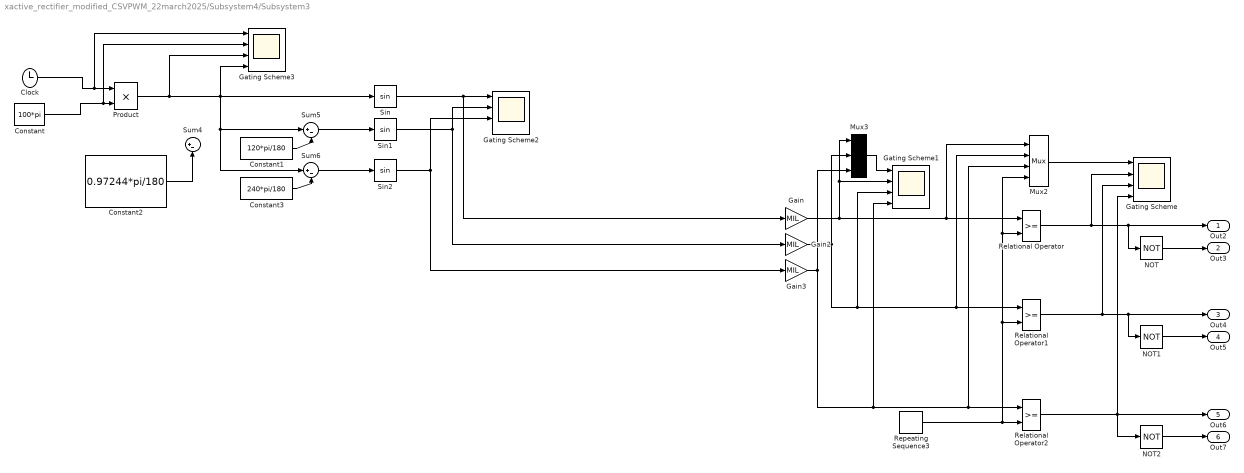
== system xactive_rectifier_modified_CSVPWM_22march2025/Subsystem4/Subsystem3 ==
  Clock : Clock
  Constant : Constant  Value=100*pi
  Constant1 : Constant  Value=120*pi/180
  Constant2 : Constant  Value=0.97244*pi/180
  Constant3 : Constant  Value=240*pi/180
  Gain : Gain  Gain=MIL
  Gain2 : Gain  Gain=MIL
  Gain3 : Gain  Gain=MIL
  Gating Scheme{,1..3} (4 alike) : Scope  NumInputPorts=4
  Mux2 : Mux
  Mux3 : Mux  Inputs=3.
  NOT : Logic  Operator=NOT  IconShape=distinctive  AllPortsSameDT=off  OutDataTypeStr=boolean
  NOT1 : Logic  Operator=NOT  IconShape=distinctive  AllPortsSameDT=off  OutDataTypeStr=boolean
  NOT2 : Logic  Operator=NOT  IconShape=distinctive  AllPortsSameDT=off  OutDataTypeStr=boolean
  Product : Product
  Relational Operator : RelationalOperator  OutDataTypeStr=boolean  RndMeth=Simplest  InputSameDT=off
  Relational Operator1 : RelationalOperator  OutDataTypeStr=boolean  RndMeth=Simplest  InputSameDT=off
  Relational Operator2 : RelationalOperator  OutDataTypeStr=boolean  RndMeth=Simplest  InputSameDT=off
  Repeating Sequence3 : simulink/Sources/Repeating Sequence  rep_seq_t=[0 1 2]*[1/10000]  rep_seq_y=[-1 1 -1]
  Sin : Trigonometry
  Sin1 : Trigonometry
  Sin2 : Trigonometry
  Sum4 : Sum  Inputs=|+-
  Sum5 : Sum  Inputs=|+-
  Sum6 : Sum  Inputs=|+-
  Out2 : Outport
  Out3 : Outport  Port=2
  Out4 : Outport  Port=3
  Out5 : Outport  Port=4
  Out6 : Outport  Port=5
  Out7 : Outport  Port=6
  wires:
  Constant2/1 -> Sum4/2
  Mux3/1 -> Gating Scheme1/1
  Gain3/1 -> Mux3/3, Relational Operator2/1, Mux2/3, Gating Scheme1/4
  Gain2/1 -> Mux3/2, Relational Operator1/1, Mux2/2, Gating Scheme1/3
  Gain/1 -> Relational Operator/1, Mux2/1, Gating Scheme1/2, Mux3/1
  NOT1/1 -> Out5/1
  Sum6/1 -> Sin2/1
  Constant3/1 -> Sum6/2
  Sin/1 -> Gating Scheme2/1, Gain/1
  Relational Operator1/1 -> Gating Scheme/3, NOT1/1, Out4/1
  Repeating Sequence3/1 -> Relational Operator2/2, Mux2/4, Relational Operator/2, Relational Operator1/2
  Clock/1 -> Product/1, Gating Scheme3/1
  Mux2/1 -> Gating Scheme/1
  Product/1 -> Gating Scheme3/3, Sum5/1, Sum6/1, Sin/1, Gating Scheme3/4
  Sum5/1 -> Sin1/1
  Sin1/1 -> Gating Scheme2/2, Gain2/1
  Relational Operator/1 -> Gating Scheme/2, NOT/1, Out2/1
  NOT/1 -> Out3/1
  Sin2/1 -> Gain3/1, Gating Scheme2/3
  Relational Operator2/1 -> NOT2/1, Gating Scheme/4, Out6/1
  Constant1/1 -> Sum5/2
  Constant/1 -> Product/2, Gating Scheme3/2
  NOT2/1 -> Out7/1
